simulink model "SST_MMC"  (R2014a)
settings: Solver=ode45  StartTime=0.0  StopTime=0.2  RelTol=1e-3
libraries: powerlib x328, simulink x1
(part 1 of 3)
settings Model: Creator=Shohag  LastModifiedBy=Shohag

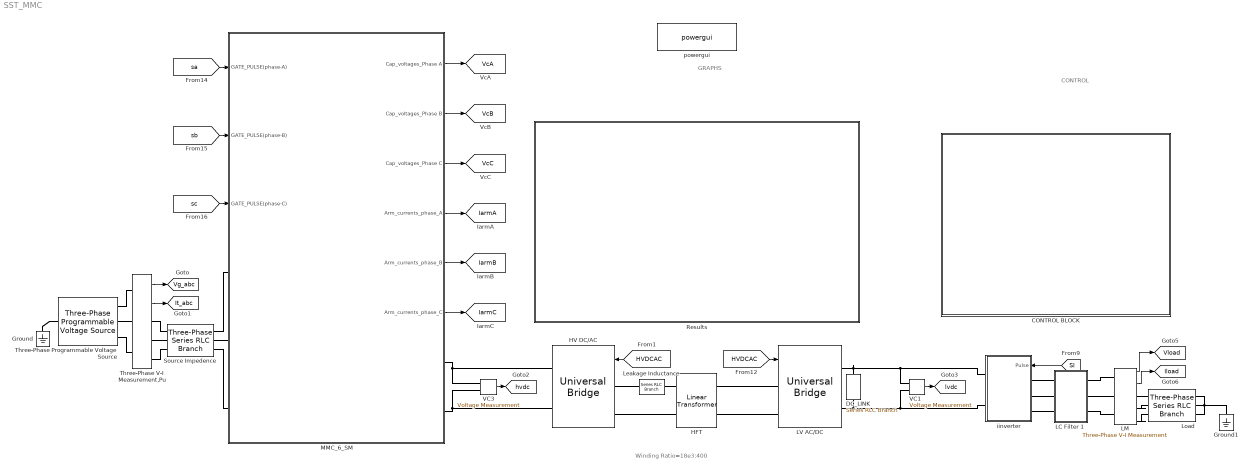
== system SST_MMC ==
  note: Winding Ratio=18e3:400
  note: GRAPHS
  note: CONTROL
  CONTROL BLOCK : Subsystem
  DC_LINK : powerlib/Elements/Series RLC Branch  LConnTagsString=__new0  RConnTagsString=__new0  BranchType=C  Resistance=1e3  Inductance=100e-6  SetiL0=off  InitialCurrent=0  Capacitance=1e-3  Setx0=off  InitialVoltage=415  Measurements=None
  Ground : powerlib/Elements/Ground  LConnTagsString=a
  Ground1 : powerlib/Elements/Ground  LConnTagsString=a
  HFT : powerlib/Elements/Linear Transformer  UNITS=pu  NominalPower=[ 10e3 10e3 ]  winding1="[ 18e3  0 0]"  winding2="[ 400  0 0]"  ThreeWindings=off  winding3=[ 315e3 0.002 0.08 ]  RmLm=[ 500e6 500e6 ]  Measurements=None  DataType=off
  HV DC/AC : powerlib/Power Electronics/Universal Bridge  Arms=2  SnubberResistance=1e5  SnubberCapacitance=inf  Device=IGBT / Diodes  Ron=1e-3  Lon=0  ForwardVoltages="[  0  0  ]"  ForwardVoltage=0  GTOparameters=[ 10e-6 , 20e-6 ]  IGBTparameters=[ 1e-6 , 2e-6 ]  Measurements=None  Measurements_2=None  converterType=Rectifier
  LC Filter 1 : Subsystem  mask{L=50e-3, C=100e-6}
      mask prompts: L "Inductance"; C "Capacitance"
  LM : powerlib/Measurements/Three-Phase V-I Measurement  VoltageMeasurement=phase-to-ground  SetLabelV=off  LabelV=Vabc  Vpu=off  VpuLL=off  CurrentMeasurement=yes  SetLabelI=off  LabelI=Iabc  Ipu=off  Pbase=20e6  Vbase=11e3  OutputType=Complex  PhasorSimulation=off  PSBequivalent=0
  LV AC/DC : powerlib/Power Electronics/Universal Bridge  Arms=2  SnubberResistance=1e5  SnubberCapacitance=inf  Device=IGBT / Diodes  Ron=1e-3  Lon=0  ForwardVoltages="[  0  0  ]"  ForwardVoltage=0  GTOparameters=[ 10e-6 , 20e-6 ]  IGBTparameters=[ 1e-6 , 2e-6 ]  Measurements=None  Measurements_2=None  converterType=Rectifier
  Leakage Inductance : powerlib/Elements/Series RLC Branch  LConnTagsString=__new0  RConnTagsString=__new0  BranchType=L  Resistance=1e3  Inductance=200e-6  SetiL0=off  InitialCurrent=0  Capacitance=0.001  Setx0=on  InitialVoltage=9e3  Measurements=None
  Load : powerlib/Elements/Three-Phase Series RLC Branch  LConnTagsString=A|B|C  RConnTagsString=A|B|C  BranchType=RL  Resistance=22  Inductance=10e-3  Capacitance=1e-6  Measurements=None
  MMC_6_SM : Subsystem  mask{C_SM=10e-3, VC_SM=3000, L_ARM=3e-3, Ron=1e-4}
      mask prompts: C_SM "Sub-module Capasitor Capasitance"; VC_SM "Sub-modue Capasitor Voltage"; L_ARM "Arm Inductance"
  Results : Subsystem
  Source Impedence : powerlib/Elements/Three-Phase Series RLC Branch  LConnTagsString=A|B|C  RConnTagsString=A|B|C  BranchType=RL  Resistance=0.5  Inductance=3e-3  Capacitance=1e-6  Measurements=None
  Three-Phase Programmable Voltage Source : powerlib/Electrical Sources/Three-Phase Programmable Voltage Source  PositiveSequence="[11e3  0 60]"  VariationEntity=Amplitude  VariationType=Table of time-amplitude pairs  VariationTypeAlt=Modulation  VariationStep=2  VariationRate=10  VariationMagnitude=0.3  VariationFrequency=5  VariationTiming=[0.1 0.2]  VariationPhaseA=on  Amplitudes=[1 0.8 1.2 0 0 1.2 1.0]  TimeValues=[0 0.03 0.05 0.07 0.08 0.09 0.1]  HarmonicGeneration=off  HarmonicA=[3 0.2 -25 0]  HarmonicB=[2 0.15 35 2]  Timing=[0.02 0.08]  BusType=PQ  Pref=10e3  Qref=0  Qmin=-inf  Qmax=inf
  Three-Phase V-I Measurement,Pu : powerlib/Measurements/Three-Phase V-I Measurement  VoltageMeasurement=phase-to-ground  SetLabelV=off  LabelV=Vabc  Vpu=off  VpuLL=off  CurrentMeasurement=yes  SetLabelI=off  LabelI=Iabc  Ipu=off  Pbase=20e6  Vbase=11e3  OutputType=Complex  PhasorSimulation=off  PSBequivalent=0
  VC1 : powerlib/Measurements/Voltage Measurement  PhasorSimulation=off  OutputType=Complex  PSBequivalent=0
  VC3 : powerlib/Measurements/Voltage Measurement  PhasorSimulation=off  OutputType=Complex  PSBequivalent=0
  iinverter : Subsystem
  powergui : powerlib/powergui  Priority=1  SimulationMode=Discrete  SolverType=Tustin  SampleTime=50e-6  frequency=60  SPID=on  DisableSnubberDevices=off  DisableRonSwitches=off  DisableVfSwitches=off  SwTol=0  Interpol=off  DisplayEquations=off  Ts=0  methode=off  frequencyindice=0  Pbase=100e6  ErrMax=1e-4  Iterations=50  UnitsV=kV  UnitsW=MW  FunctionMessages=off  echomessages=off  HookPort=off  EnableUseOfTLC=off  x0status=blocks  RestoreLinks=warning  ResistiveCurrentMeasurement=off  Frange=[0:2:500]  Ylog=off  Xlog=on  ShowGrid=off  save=off  variable=ZData  structure=0  ZoomFFT=off  StartTime=0.0  cycles=1  DisplayStyle=1  fundamental=60  FreqAxis=off  MaxFrequency=1000  frequencyindicesteady=1  RmsSteady=2  display=off
  tag scope: IarmA=global, IarmB=global, IarmC=global, Iload=global, It_abc=global, VcA=global, VcB=global, VcC=global, Vg_abc=global, Vload=global, hvdc=global, lvdc=global
  wires:
  MMC_6_SM/1(Cap_voltages_Phase A) -> [VcA]
  MMC_6_SM/2(Cap_voltages_Phase B) -> [VcB]
  MMC_6_SM/3(Cap_voltages_Phase C) -> [VcC]
  MMC_6_SM/4(Arm_currents_phase_A) -> [IarmA]
  MMC_6_SM/5(Arm_currents_phase_B) -> [IarmB]
  MMC_6_SM/6(Arm_currents_phase_C) -> [IarmC]
  Three-Phase V-I Measurement,Pu/1 -> [Vg_abc]
  Three-Phase V-I Measurement,Pu/2 -> [It_abc]
  VC3/1 -> [hvdc]
  [sa] -> MMC_6_SM/1(" GATE_PULSE(phase-A) ")
  [sb] -> MMC_6_SM/2(" GATE_PULSE(phase-B) ")
  [sc] -> MMC_6_SM/3(" GATE_PULSE(phase-C) ")
  VC1/1 -> [lvdc]
  [HVDCAC] -> HV DC/AC/1
  [HVDCAC] -> LV AC/DC/1
  [SI] -> iinverter/1(Pulse)
  LM/1 -> [Vload]
  LM/2 -> [Iload]
  connections:
  Source Impedence/RConn1 -- MMC_6_SM/LConn1
  Source Impedence/RConn2 -- MMC_6_SM/LConn2
  Three-Phase Programmable Voltage Source/RConn3 -- Three-Phase V-I Measurement,Pu/LConn3
  Three-Phase Programmable Voltage Source/RConn1 -- Three-Phase V-I Measurement,Pu/LConn1
  Three-Phase Programmable Voltage Source/RConn2 -- Three-Phase V-I Measurement,Pu/LConn2
  Three-Phase V-I Measurement,Pu/RConn3 -- Source Impedence/LConn3
  Three-Phase Programmable Voltage Source/LConn1 -- Ground/LConn1
  Three-Phase V-I Measurement,Pu/RConn1 -- Source Impedence/LConn1
  Source Impedence/RConn3 -- MMC_6_SM/LConn3
  Three-Phase V-I Measurement,Pu/RConn2 -- Source Impedence/LConn2
  HV DC/AC/LConn2 -- HFT/LConn2
  LV AC/DC/LConn1 -- HFT/RConn1
  LV AC/DC/LConn2 -- HFT/RConn2
  VC3/LConn2 -- HV DC/AC/RConn2 -- MMC_6_SM/RConn2
  HV DC/AC/LConn1 -- Leakage Inductance/RConn1
  VC1/LConn2 -- iinverter/RConn2 -- DC_LINK/RConn1 -- LV AC/DC/RConn2
  Leakage Inductance/LConn1 -- HFT/LConn1
  VC3/LConn1 -- HV DC/AC/RConn1 -- MMC_6_SM/RConn1
  VC1/LConn1 -- DC_LINK/LConn1 -- LV AC/DC/RConn1 -- iinverter/RConn1
  Load/RConn1 -- Ground1/LConn1 -- Load/RConn3 -- Load/RConn2
  LM/RConn1 -- Load/LConn1
  LM/RConn2 -- Load/LConn2
  LM/RConn3 -- Load/LConn3
  iinverter/LConn3 -- LC Filter 1/LConn3
  iinverter/LConn2 -- LC Filter 1/LConn2
  iinverter/LConn1 -- LC Filter 1/LConn1
  LC Filter 1/RConn1 -- LM/LConn1
  LC Filter 1/RConn2 -- LM/LConn2
  LC Filter 1/RConn3 -- LM/LConn3

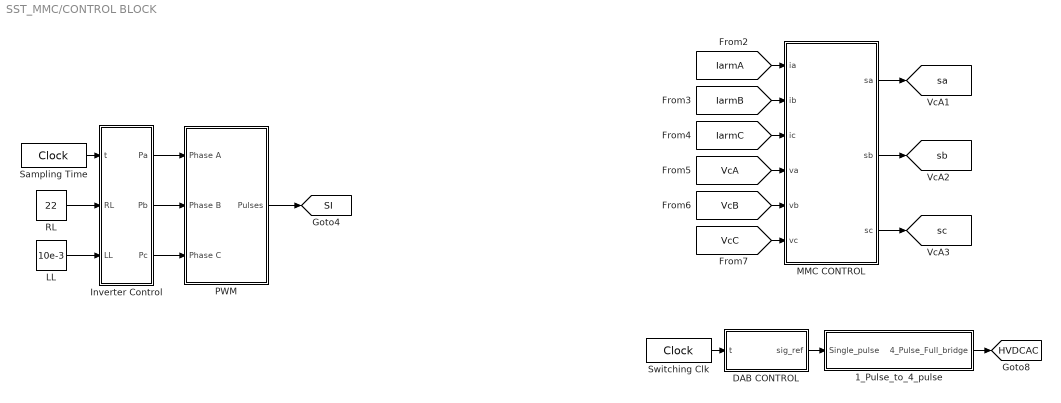
== system SST_MMC/CONTROL BLOCK ==
  1_Pulse_to_4_pulse : Subsystem
  DAB CONTROL : MATLAB Function  TreatAsAtomicUnit=on
  Inverter Control : MATLAB Function  TreatAsAtomicUnit=on
  LL : Constant  Value=10e-3
  MMC CONTROL : MATLAB Function  TreatAsAtomicUnit=on
  PWM : Subsystem  mask{Fs=10e3}
      mask prompts: Fs "Frequency"
  RL : Constant  Value=22
  Sampling Time : DigitalClock  SampleTime=100e-6
  Switching Clk : DigitalClock  SampleTime=5e-5
  tag scope: HVDCAC=global, SI=global, sa=global, sb=global, sc=global
  wires:
  LL/1 -> Inverter Control/3(LL)
  RL/1 -> Inverter Control/2(RL)
  Inverter Control/1(Pa) -> PWM/1(Phase A)
  Inverter Control/2(Pb) -> PWM/2(Phase B)
  Inverter Control/3(Pc) -> PWM/3(Phase C)
  PWM/1(Pulses) -> [SI]
  Switching Clk/1 -> DAB CONTROL/1(t)
  MMC CONTROL/3(sc) -> [sc]
  MMC CONTROL/2(sb) -> [sb]
  MMC CONTROL/1(sa) -> [sa]
  1_Pulse_to_4_pulse/1(4_Pulse_Full_bridge) -> [HVDCAC]
  DAB CONTROL/1(sig_ref) -> 1_Pulse_to_4_pulse/1(Single_pulse)
  Sampling Time/1 -> Inverter Control/1(t)
  [VcA] -> MMC CONTROL/4(va)
  [IarmC] -> MMC CONTROL/3(ic)
  [IarmB] -> MMC CONTROL/2(ib)
  [VcC] -> MMC CONTROL/6(vc)
  [IarmA] -> MMC CONTROL/1(ia)
  [VcB] -> MMC CONTROL/5(vb)

== system SST_MMC/LC Filter 1 ==
  C5 : powerlib/Elements/Parallel RLC Branch  LConnTagsString=a  RConnTagsString=__new0  BranchType=C  Resistance=inf  Inductance=inf  SetiL0=off  InitialCurrent=0  Capacitance=C  Setx0=off  InitialVoltage=0  Measurements=None
  C6 : powerlib/Elements/Parallel RLC Branch  LConnTagsString=a  RConnTagsString=__new0  BranchType=C  Resistance=inf  Inductance=inf  SetiL0=off  InitialCurrent=0  Capacitance=C  Setx0=off  InitialVoltage=0  Measurements=None
  C7 : powerlib/Elements/Parallel RLC Branch  LConnTagsString=a  RConnTagsString=__new0  BranchType=C  Resistance=inf  Inductance=inf  SetiL0=off  InitialCurrent=0  Capacitance=C  Setx0=off  InitialVoltage=0  Measurements=None
  Ground2 : powerlib/Elements/Ground  LConnTagsString=a
  L4 : powerlib/Elements/Parallel RLC Branch  LConnTagsString=a  RConnTagsString=__new0  BranchType=L  Resistance=inf  Inductance=L  SetiL0=off  InitialCurrent=0  Capacitance=1.3e-3  Setx0=off  InitialVoltage=0  Measurements=None
  L5 : powerlib/Elements/Parallel RLC Branch  LConnTagsString=a  RConnTagsString=__new0  BranchType=L  Resistance=inf  Inductance=L  SetiL0=off  InitialCurrent=0  Capacitance=1.3e-3  Setx0=off  InitialVoltage=0  Measurements=None
  L6 : powerlib/Elements/Parallel RLC Branch  LConnTagsString=a  RConnTagsString=__new0  BranchType=L  Resistance=inf  Inductance=L  SetiL0=off  InitialCurrent=0  Capacitance=1.3e-3  Setx0=off  InitialVoltage=0  Measurements=None
  A : PMIOPort  Port=1  Side=Left
  A1 : PMIOPort  Port=2  Side=Right
  B : PMIOPort  Port=3  Side=Left
  B1 : PMIOPort  Port=4  Side=Right
  C1 : PMIOPort  Port=5  Side=Right
  C : PMIOPort  Port=6  Side=Left
  connections:
  L4/LConn1 -- A/RConn1
  L6/LConn1 -- C/RConn1
  C5/RConn1 -- C7/RConn1 -- Ground2/LConn1 -- C6/RConn1
  L5/LConn1 -- B/RConn1
  C6/LConn1 -- B1/RConn1 -- L5/RConn1
  L4/RConn1 -- A1/RConn1 -- C5/LConn1
  C7/LConn1 -- C1/RConn1 -- L6/RConn1

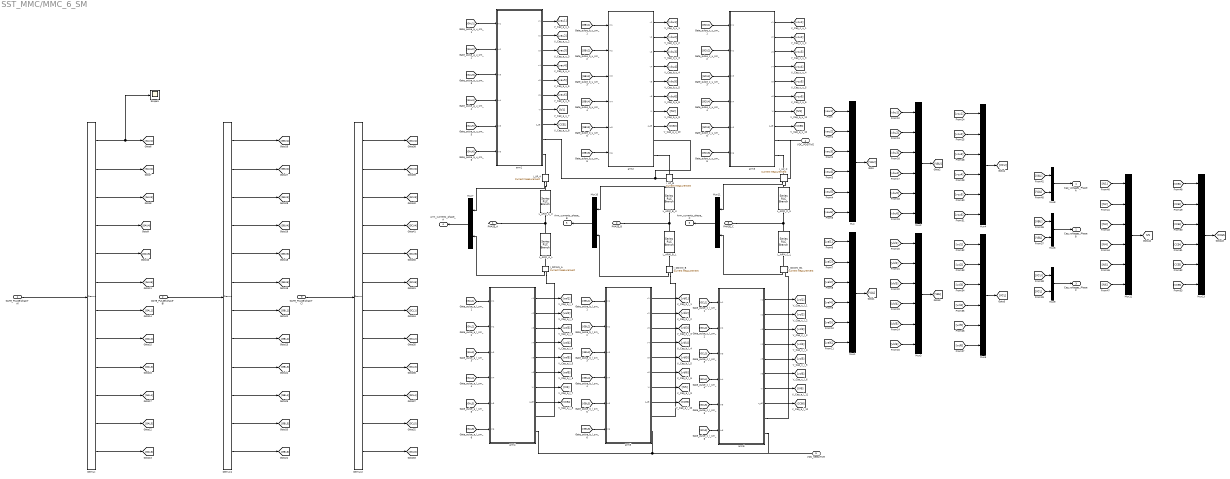
== system SST_MMC/MMC_6_SM ==
  " GATE_PULSE(phase-A) " : Inport
  " GATE_PULSE(phase-B) " : Inport  Port=2
  " GATE_PULSE(phase-C) " : Inport  Port=3
  Demux : Demux  Outputs=12
  Demux1 : Demux  Outputs=12
  Demux2 : Demux  Outputs=12
  I_DOWN_A : powerlib/Measurements/Current Measurement  PhasorSimulation=off  OutputType=Complex  PSBequivalent=0
  I_DOWN_B : powerlib/Measurements/Current Measurement  PhasorSimulation=off  OutputType=Complex  PSBequivalent=0
  I_DOWN_B1 : powerlib/Measurements/Current Measurement  PhasorSimulation=off  OutputType=Complex  PSBequivalent=0
  I_UP_A : powerlib/Measurements/Current Measurement  PhasorSimulation=off  OutputType=Complex  PSBequivalent=0
  I_UP_B : powerlib/Measurements/Current Measurement  PhasorSimulation=off  OutputType=Complex  PSBequivalent=0
  I_UP_C : powerlib/Measurements/Current Measurement  PhasorSimulation=off  OutputType=Complex  PSBequivalent=0
  L_ARM_A_L : powerlib/Elements/Series RLC Branch  LConnTagsString=__new0  RConnTagsString=__new0  BranchType=L  Resistance=1  Inductance=L_ARM  SetiL0=off  InitialCurrent=0  Capacitance=1e-6  Setx0=off  InitialVoltage=0  Measurements=None
  L_ARM_A_U : powerlib/Elements/Series RLC Branch  LConnTagsString=__new0  RConnTagsString=__new0  BranchType=L  Resistance=1  Inductance=L_ARM  SetiL0=off  InitialCurrent=0  Capacitance=1e-6  Setx0=off  InitialVoltage=0  Measurements=None
  L_ARM_B_L : powerlib/Elements/Series RLC Branch  LConnTagsString=__new0  RConnTagsString=__new0  BranchType=L  Resistance=1  Inductance=L_ARM  SetiL0=off  InitialCurrent=0  Capacitance=1e-6  Setx0=off  InitialVoltage=0  Measurements=None
  L_ARM_B_U : powerlib/Elements/Series RLC Branch  LConnTagsString=__new0  RConnTagsString=__new0  BranchType=L  Resistance=1  Inductance=L_ARM  SetiL0=off  InitialCurrent=0  Capacitance=1e-6  Setx0=off  InitialVoltage=0  Measurements=None
  L_ARM_C_L : powerlib/Elements/Series RLC Branch  LConnTagsString=__new0  RConnTagsString=__new0  BranchType=L  Resistance=1  Inductance=L_ARM  SetiL0=off  InitialCurrent=0  Capacitance=1e-6  Setx0=off  InitialVoltage=0  Measurements=None
  L_ARM_C_U : powerlib/Elements/Series RLC Branch  LConnTagsString=__new0  RConnTagsString=__new0  BranchType=L  Resistance=1  Inductance=L_ARM  SetiL0=off  InitialCurrent=0  Capacitance=1e-6  Setx0=off  InitialVoltage=0  Measurements=None
  Mux{,1..5,12..13} (8 alike) : Mux  Inputs=6
  Mux{6..11} (6 alike) : Mux  Inputs=2
  Scope1 : Scope
      settings: YMin=0.95  YMax=1.05  SaveName=ScopeData3
  arm1 : Subsystem
  arm2 : Subsystem
  arm3 : Subsystem
  arm4 : Subsystem
  arm5 : Subsystem
  arm6 : Subsystem
  PHASE_A : PMIOPort  Port=1  Side=Left
  PHASE_B : PMIOPort  Port=2  Side=Left
  PHASE_C : PMIOPort  Port=3  Side=Left
  VDC_POSITIVE : PMIOPort  Port=4  Side=Right
  VDC_NEGATIVE : PMIOPort  Port=5  Side=Right
  Cap_voltages_Phase A : Outport
  Cap_voltages_Phase B : Outport  Port=2
  Cap_voltages_Phase C : Outport  Port=3
  Arm_currents_phase_A : Outport  Port=4
  Arm_currents_phase_B : Outport  Port=5
  Arm_currents_phase_C : Outport  Port=6
  tag scope: CCES=global, IVS=global
  wires:
  Demux/4 -> [GAU4]
  Demux/2 -> [GAU2]
  [vau2] -> Mux/2
  [vau1] -> Mux/1
  Mux/1 -> [VAU]
  Demux/1 -> Scope1/1, [GAU1]
  [vbl6] -> Mux3/6
  [vbl4] -> Mux3/4
  [vbu6] -> Mux2/6
  [vbu1] -> Mux2/1
  [vbu4] -> Mux2/4
  [vbl3] -> Mux3/3
  Mux2/1 -> [VBU]
  [vbu3] -> Mux2/3
  [vbl1] -> Mux3/1
  Mux3/1 -> [VBL]
  [vbu5] -> Mux2/5
  [vbu2] -> Mux2/2
  [vbl2] -> Mux3/2
  [vbl5] -> Mux3/5
  Demux1/1 -> [GBU1]
  Demux1/3 -> [GBU3]
  [vcl6] -> Mux5/6
  [vcl5] -> Mux5/5
  [vcu3] -> Mux4/3
  [vcl1] -> Mux5/1
  [vcl4] -> Mux5/4
  [vcu5] -> Mux4/5
  [vcu2] -> Mux4/2
  [vcl3] -> Mux5/3
  Mux4/1 -> [VCU]
  [vcu6] -> Mux4/6
  Mux5/1 -> [VCL]
  [vcl2] -> Mux5/2
  [vcu1] -> Mux4/1
  [vcu4] -> Mux4/4
  [vau3] -> Mux/3
  [val5] -> Mux1/5
  Demux/3 -> [GAU3]
  Demux/5 -> [GAU5]
  [vau6] -> Mux/6
  [val4] -> Mux1/4
  Mux1/1 -> [VAL]
  [vau4] -> Mux/4
  [val3] -> Mux1/3
  [val6] -> Mux1/6
  [val2] -> Mux1/2
  Demux/6 -> [GAU6]
  [vau5] -> Mux/5
  [val1] -> Mux1/1
  Mux7/1 -> Arm_currents_phase_A/1
  [VAL] -> Mux8/2
  [VAU] -> Mux8/1
  Mux8/1 -> Cap_voltages_Phase A/1
  Demux/7 -> [GAL1]
  Demux/8 -> [GAL2]
  Demux/9 -> [GAL3]
  Demux/10 -> [GAL4]
  Demux/11 -> [GAL5]
  Demux/12 -> [GAL6]
  Demux1/2 -> [GBU2]
  Demux1/4 -> [GBU4]
  Demux1/5 -> [GBU5]
  Demux1/6 -> [GBU6]
  Demux1/7 -> [GBL1]
  Demux1/8 -> [GBL2]
  Demux1/9 -> [GBL3]
  Demux1/10 -> [GBL4]
  Demux1/11 -> [GBL5]
  Demux1/12 -> [GBL6]
  Demux2/1 -> [GCU1]
  Demux2/2 -> [GCU2]
  Demux2/3 -> [GCU3]
  Demux2/4 -> [GCU4]
  Demux2/5 -> [GCU5]
  Demux2/6 -> [GCU6]
  Demux2/7 -> [GCL1]
  Demux2/8 -> [GCL2]
  Demux2/9 -> [GCL3]
  Demux2/10 -> [GCL4]
  Demux2/11 -> [GCL5]
  Demux2/12 -> [GCL6]
  [VBL] -> Mux6/2
  [VBU] -> Mux6/1
  Mux6/1 -> Cap_voltages_Phase B/1
  [VCL] -> Mux9/2
  [VCU] -> Mux9/1
  Mux9/1 -> Cap_voltages_Phase C/1
  Mux10/1 -> Arm_currents_phase_B/1
  I_DOWN_B/1 -> Mux10/2
  Mux11/1 -> Arm_currents_phase_C/1
  I_DOWN_B1/1 -> Mux11/2
  I_UP_A/1 -> Mux7/1
  I_DOWN_A/1 -> Mux7/2
  I_UP_B/1 -> Mux10/1
  I_UP_C/1 -> Mux11/1
  " GATE_PULSE(phase-A) "/1 -> Demux/1
  " GATE_PULSE(phase-B) "/1 -> Demux1/1
  " GATE_PULSE(phase-C) "/1 -> Demux2/1
  [GAU6] -> arm1/6(In6)
  [GAU5] -> arm1/5(In5)
  [GAU4] -> arm1/4(In4)
  [GAU3] -> arm1/3(In3)
  [GAU2] -> arm1/2(In2)
  [GAU1] -> arm1/1(In1)
  arm1/1(v1) -> [vau1]
  arm1/2(v2) -> [vau2]
  arm1/3(v3) -> [vau3]
  arm1/4(v4) -> [vau4]
  arm1/5(v5) -> [vau5]
  arm1/6(v6) -> [vau6]
  [GBU6] -> arm2/6(In6)
  [GBU5] -> arm2/5(In5)
  [GBU4] -> arm2/4(In4)
  [GBU3] -> arm2/3(In3)
  [GBU2] -> arm2/2(In2)
  [GBU1] -> arm2/1(In1)
  arm2/1(v1) -> [vbu1]
  arm2/2(v2) -> [vbu2]
  arm2/3(v3) -> [vbu3]
  arm2/4(v4) -> [vbu4]
  arm2/5(v5) -> [vbu5]
  arm2/6(v6) -> [vbu6]
  arm1/7(VI) -> [IV1]
  arm1/8(c_cE) -> [CCE1]
  arm2/7(VI) -> [IV2]
  arm2/8(c_cE) -> [CCE2]
  [GCU6] -> arm3/6(In6)
  [GCU5] -> arm3/5(In5)
  [GCU4] -> arm3/4(In4)
  [GCU3] -> arm3/3(In3)
  [GCU2] -> arm3/2(In2)
  [GCU1] -> arm3/1(In1)
  arm3/1(v1) -> [vcu1]
  arm3/2(v2) -> [vcu2]
  arm3/3(v3) -> [vcu3]
  arm3/4(v4) -> [vcu4]
  arm3/5(v5) -> [vcu5]
  arm3/6(v6) -> [vcu6]
  arm3/7(VI) -> [IV3]
  arm3/8(c_cE) -> [CCE3]
  [GAL1] -> arm4/1(In1)
  [GAL2] -> arm4/2(In2)
  [GAL3] -> arm4/3(In3)
  [GAL4] -> arm4/4(In4)
  [GAL5] -> arm4/5(In5)
  [GAL6] -> arm4/6(In6)
  arm4/1(v1) -> [val1]
  arm4/2(v2) -> [val2]
  arm4/3(v3) -> [val3]
  arm4/4(v4) -> [val4]
  arm4/5(v5) -> [val5]
  arm4/6(v6) -> [val6]
  arm4/7(VI) -> [IV4]
  arm4/8(c_cE) -> [CCE4]
  [GBL1] -> arm5/1(In1)
  [GBL2] -> arm5/2(In2)
  [GBL3] -> arm5/3(In3)
  [GBL4] -> arm5/4(In4)
  [GBL5] -> arm5/5(In5)
  [GBL6] -> arm5/6(In6)
  arm5/1(v1) -> [vbl1]
  arm5/2(v2) -> [vbl2]
  arm5/3(v3) -> [vbl3]
  arm5/4(v4) -> [vbl4]
  arm5/5(v5) -> [vbl5]
  arm5/6(v6) -> [vbl6]
  arm5/7(VI) -> [IV5]
  arm5/8(c_cE) -> [CCE5]
  [GCL1] -> arm6/1(In1)
  [GCL2] -> arm6/2(In2)
  [GCL3] -> arm6/3(In3)
  [GCL4] -> arm6/4(In4)
  [GCL5] -> arm6/5(In5)
  [GCL6] -> arm6/6(In6)
  arm6/1(v1) -> [vcl1]
  arm6/2(v2) -> [vcl2]
  arm6/3(v3) -> [vcl3]
  arm6/4(v4) -> [vcl4]
  arm6/5(v5) -> [vcl5]
  arm6/6(v6) -> [vcl6]
  arm6/7(VI) -> [IV6]
  arm6/8(c_cE) -> [CCE6]
  [IV5] -> Mux12/5
  [IV2] -> Mux12/2
  Mux12/1 -> [IVS]
  [IV6] -> Mux12/6
  [IV1] -> Mux12/1
  [IV4] -> Mux12/4
  [CCE3] -> Mux13/3
  [CCE5] -> Mux13/5
  [CCE2] -> Mux13/2
  Mux13/1 -> [CCES]
  [CCE6] -> Mux13/6
  [CCE1] -> Mux13/1
  [CCE4] -> Mux13/4
  [IV3] -> Mux12/3
  connections:
  L_ARM_A_U/RConn1 -- PHASE_A/RConn1 -- L_ARM_A_L/LConn1
  L_ARM_B_U/RConn1 -- PHASE_B/RConn1 -- L_ARM_B_L/LConn1
  L_ARM_C_U/RConn1 -- PHASE_C/RConn1 -- L_ARM_C_L/LConn1
  L_ARM_B_L/RConn1 -- I_DOWN_B/LConn1
  L_ARM_C_L/RConn1 -- I_DOWN_B1/LConn1
  I_UP_A/RConn1 -- L_ARM_A_U/LConn1
  I_DOWN_A/LConn1 -- L_ARM_A_L/RConn1
  I_UP_B/RConn1 -- L_ARM_B_U/LConn1
  I_UP_C/RConn1 -- L_ARM_C_U/LConn1
  arm1/RConn1 -- arm2/RConn1 -- VDC_POSITIVE/RConn1 -- arm3/RConn1
  I_DOWN_A/RConn1 -- arm4/RConn1
  I_DOWN_B/RConn1 -- arm5/RConn1
  arm4/RConn2 -- arm6/RConn2 -- VDC_NEGATIVE/RConn1 -- arm5/RConn2
  arm6/RConn1 -- I_DOWN_B1/RConn1
  arm1/RConn2 -- I_UP_A/LConn1
  arm2/RConn2 -- I_UP_B/LConn1
  arm3/RConn2 -- I_UP_C/LConn1

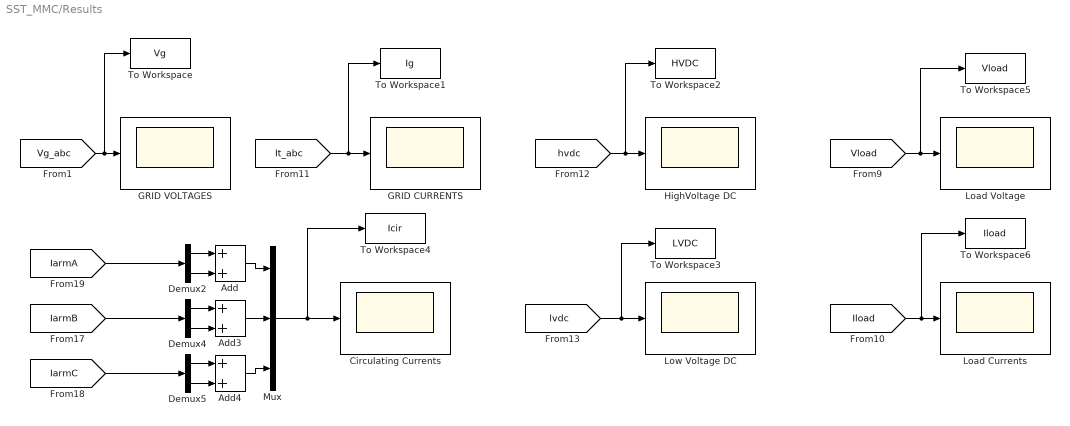
== system SST_MMC/Results ==
  Add : Sum
  Add3 : Sum
  Add4 : Sum
  Circulating Currents : Scope
      settings: YMin=-30  YMax=40  SaveName=ScopeData5
  Demux2 : Demux  Outputs=2
  Demux4 : Demux  Outputs=2
  Demux5 : Demux  Outputs=2
  GRID CURRENTS : Scope
      settings: YMin=-20000  YMax=20000  SaveName=ScopeData4
  GRID VOLTAGES : Scope
      settings: YMin=-17500  YMax=17500
  HighVoltage DC : Scope
      settings: YMin=15500  YMax=20500  SaveName=ScopeData6
  Load Currents : Scope
      settings: YMin=-25  YMax=35  SaveName=ScopeData10
  Load Voltage : Scope
      settings: YMin=-300  YMax=300  SaveName=ScopeData9
  Low Voltage DC : Scope
      settings: YMin=427.75  YMax=432.25  SaveName=ScopeData8
  Mux : Mux  Inputs=3
  To Workspace : ToWorkspace  VariableName=Vg  SaveFormat=Timeseries  SampleTime=-1
  To Workspace1 : ToWorkspace  VariableName=Ig  SaveFormat=Timeseries  SampleTime=-1
  To Workspace2 : ToWorkspace  VariableName=HVDC  SaveFormat=Timeseries  SampleTime=-1
  To Workspace3 : ToWorkspace  VariableName=LVDC  SaveFormat=Timeseries  SampleTime=-1
  To Workspace4 : ToWorkspace  VariableName=Icir  SaveFormat=Timeseries  SampleTime=-1
  To Workspace5 : ToWorkspace  VariableName=Vload  SaveFormat=Timeseries  SampleTime=-1
  To Workspace6 : ToWorkspace  VariableName=Iload  SaveFormat=Timeseries  SampleTime=-1
  wires:
  [hvdc] -> To Workspace2/1, HighVoltage DC/1
  Add4/1 -> Mux/3
  [IarmA] -> Demux2/1
  Demux2/1 -> Add/1
  Demux2/2 -> Add/2
  [Vg_abc] -> To Workspace/1, GRID VOLTAGES/1
  Demux4/2 -> Add3/2
  [IarmB] -> Demux4/1
  Demux5/1 -> Add4/1
  Mux/1 -> To Workspace4/1, Circulating Currents/1
  Add3/1 -> Mux/2
  Demux5/2 -> Add4/2
  Add/1 -> Mux/1
  [lvdc] -> To Workspace3/1, Low Voltage DC/1
  Demux4/1 -> Add3/1
  [IarmC] -> Demux5/1
  [It_abc] -> To Workspace1/1, GRID CURRENTS/1
  [Vload] -> To Workspace5/1, Load Voltage/1
  [Iload] -> To Workspace6/1, Load Currents/1

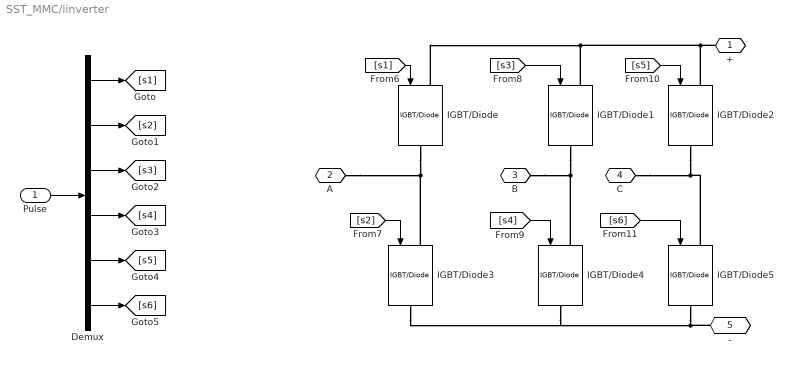
== system SST_MMC/iinverter ==
  Pulse : Inport
  Demux : Demux  Outputs=6
  IGBT/Diode{,1..5} (6 alike) : powerlib/Power Electronics/IGBT//Diode  Ron=1e-3  Rs=1e5  Cs=inf  Measurements=off
  + : PMIOPort  Port=1  Side=Right
  A : PMIOPort  Port=2  Side=Left
  B : PMIOPort  Port=3  Side=Left
  C : PMIOPort  Port=4  Side=Left
  - : PMIOPort  Port=5  Side=Right
  wires:
  [s1] -> IGBT/Diode/1
  [s2] -> IGBT/Diode3/1
  [s3] -> IGBT/Diode1/1
  [s4] -> IGBT/Diode4/1
  [s5] -> IGBT/Diode2/1
  [s6] -> IGBT/Diode5/1
  Demux/1 -> [s1]
  Demux/2 -> [s2]
  Demux/3 -> [s3]
  Demux/4 -> [s4]
  Demux/5 -> [s5]
  Demux/6 -> [s6]
  Pulse/1 -> Demux/1
  connections:
  +/RConn1 -- IGBT/Diode/LConn1 -- IGBT/Diode1/LConn1 -- IGBT/Diode2/LConn1
  IGBT/Diode4/RConn1 -- IGBT/Diode3/RConn1 -- IGBT/Diode5/RConn1 -- -/RConn1
  A/RConn1 -- IGBT/Diode3/LConn1 -- IGBT/Diode/RConn1
  B/RConn1 -- IGBT/Diode4/LConn1 -- IGBT/Diode1/RConn1
  C/RConn1 -- IGBT/Diode5/LConn1 -- IGBT/Diode2/RConn1

== system SST_MMC/CONTROL BLOCK/1_Pulse_to_4_pulse ==
  Single_pulse : Inport
  Mux1 : Mux
  Relay4 : Relay
  Relay5 : Relay  OnOutputValue=0  OffOutputValue=1
  Relay6 : Relay  OnOutputValue=0  OffOutputValue=1
  Relay7 : Relay
  4_Pulse_Full_bridge : Outport
  wires:
  Single_pulse/1 -> Relay5/1, Relay4/1, Relay7/1, Relay6/1
  Mux1/1 -> 4_Pulse_Full_bridge/1
  Relay6/1 -> Mux1/3
  Relay4/1 -> Mux1/1
  Relay7/1 -> Mux1/4
  Relay5/1 -> Mux1/2

== system SST_MMC/CONTROL BLOCK/PWM ==
  Phase A : Inport
  Phase B : Inport  Port=2
  Phase C : Inport  Port=3
  BL1 : Logic  Operator=NOT  Inputs=1
  BL2 : Logic  Operator=NOT  Inputs=1
  BL5 : Logic  Operator=NOT  Inputs=1
  Mux : Mux  Inputs=6
  Relational Operator1 : RelationalOperator  Operator=<=
  Relational Operator2 : RelationalOperator  Operator=<=
  Relational Operator3 : RelationalOperator  Operator=<=
  Triangle : simulink/Sources/Repeating Sequence  rep_seq_t=[0 1/Fs/4 3/Fs/4 1/Fs]  rep_seq_y=[0 -1 1 0]
  Pulses : Outport
  wires:
  Relational Operator3/1 -> Mux/5, BL2/1
  Triangle/1 -> Relational Operator3/1, Relational Operator1/1, Relational Operator2/1
  BL2/1 -> Mux/6
  BL5/1 -> Mux/2
  Mux/1 -> Pulses/1
  Relational Operator2/1 -> Mux/1, BL5/1
  Relational Operator1/1 -> Mux/3, BL1/1
  Phase C/1 -> Relational Operator3/2
  Phase A/1 -> Relational Operator2/2
  Phase B/1 -> Relational Operator1/2
  BL1/1 -> Mux/4

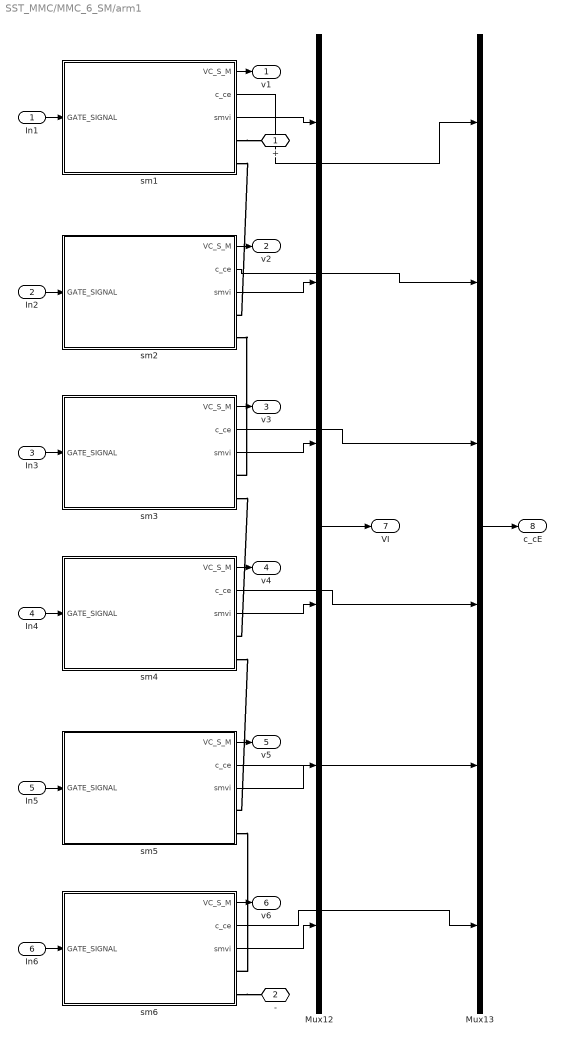
== system SST_MMC/MMC_6_SM/arm1 ==
  In1 : Inport
  In2 : Inport  Port=2
  In3 : Inport  Port=3
  In4 : Inport  Port=4
  In5 : Inport  Port=5
  In6 : Inport  Port=6
  Mux12 : Mux  Inputs=6
  Mux13 : Mux  Inputs=6
  sm1 : Subsystem
  sm2 : Subsystem
  sm3 : Subsystem
  sm4 : Subsystem
  sm5 : Subsystem
  sm6 : Subsystem
  + : PMIOPort  Port=1  Side=Right
  - : PMIOPort  Port=2  Side=Right
  v1 : Outport
  v2 : Outport  Port=2
  v3 : Outport  Port=3
  v4 : Outport  Port=4
  v5 : Outport  Port=5
  v6 : Outport  Port=6
  VI : Outport  Port=7
  c_cE : Outport  Port=8
  wires:
  sm4/2(" c_ce") -> Mux13/4
  sm5/3(" smvi") -> Mux12/5
  sm3/1(" VC_S_M") -> v3/1
  Mux13/1 -> c_cE/1
  In5/1 -> sm5/1(" GATE_SIGNAL ")
  In4/1 -> sm4/1(" GATE_SIGNAL ")
  sm5/1(" VC_S_M") -> v5/1
  In3/1 -> sm3/1(" GATE_SIGNAL ")
  sm6/1(" VC_S_M") -> v6/1
  In2/1 -> sm2/1(" GATE_SIGNAL ")
  sm2/3(" smvi") -> Mux12/2
  In1/1 -> sm1/1(" GATE_SIGNAL ")
  sm2/1(" VC_S_M") -> v2/1
  In6/1 -> sm6/1(" GATE_SIGNAL ")
  sm4/3(" smvi") -> Mux12/4
  sm1/1(" VC_S_M") -> v1/1
  sm4/1(" VC_S_M") -> v4/1
  Mux12/1 -> VI/1
  sm5/2(" c_ce") -> Mux13/5
  sm6/3(" smvi") -> Mux12/6
  sm3/2(" c_ce") -> Mux13/3
  sm1/2(" c_ce") -> Mux13/1
  sm2/2(" c_ce") -> Mux13/2
  sm3/3(" smvi") -> Mux12/3
  sm6/2(" c_ce") -> Mux13/6
  sm1/3(" smvi") -> Mux12/1
  connections:
  sm6/RConn2 -- -/RConn1
  sm1/RConn2 -- sm2/RConn1
  sm1/RConn1 -- +/RConn1
  sm2/RConn2 -- sm3/RConn1
  sm4/RConn2 -- sm5/RConn1
  sm5/RConn2 -- sm6/RConn1
  sm3/RConn2 -- sm4/RConn1

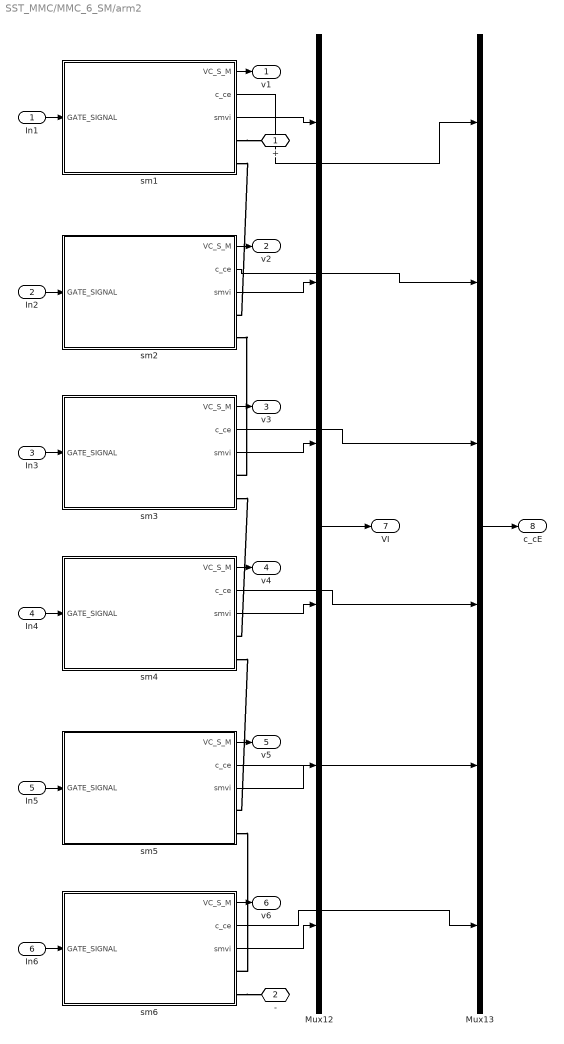
== system SST_MMC/MMC_6_SM/arm2 ==
  In1 : Inport
  In2 : Inport  Port=2
  In3 : Inport  Port=3
  In4 : Inport  Port=4
  In5 : Inport  Port=5
  In6 : Inport  Port=6
  Mux12 : Mux  Inputs=6
  Mux13 : Mux  Inputs=6
  sm1 : Subsystem
  sm2 : Subsystem
  sm3 : Subsystem
  sm4 : Subsystem
  sm5 : Subsystem
  sm6 : Subsystem
  + : PMIOPort  Port=1  Side=Right
  - : PMIOPort  Port=2  Side=Right
  v1 : Outport
  v2 : Outport  Port=2
  v3 : Outport  Port=3
  v4 : Outport  Port=4
  v5 : Outport  Port=5
  v6 : Outport  Port=6
  VI : Outport  Port=7
  c_cE : Outport  Port=8
  wires:
  sm1/3(" smvi") -> Mux12/1
  sm6/2(" c_ce") -> Mux13/6
  sm3/3(" smvi") -> Mux12/3
  sm2/2(" c_ce") -> Mux13/2
  sm1/2(" c_ce") -> Mux13/1
  sm3/2(" c_ce") -> Mux13/3
  sm6/3(" smvi") -> Mux12/6
  sm5/2(" c_ce") -> Mux13/5
  Mux12/1 -> VI/1
  sm4/1(" VC_S_M") -> v4/1
  sm1/1(" VC_S_M") -> v1/1
  sm4/3(" smvi") -> Mux12/4
  In6/1 -> sm6/1(" GATE_SIGNAL ")
  sm2/1(" VC_S_M") -> v2/1
  In1/1 -> sm1/1(" GATE_SIGNAL ")
  sm2/3(" smvi") -> Mux12/2
  In2/1 -> sm2/1(" GATE_SIGNAL ")
  sm6/1(" VC_S_M") -> v6/1
  In3/1 -> sm3/1(" GATE_SIGNAL ")
  sm5/1(" VC_S_M") -> v5/1
  In4/1 -> sm4/1(" GATE_SIGNAL ")
  In5/1 -> sm5/1(" GATE_SIGNAL ")
  Mux13/1 -> c_cE/1
  sm3/1(" VC_S_M") -> v3/1
  sm5/3(" smvi") -> Mux12/5
  sm4/2(" c_ce") -> Mux13/4
  connections:
  sm3/RConn2 -- sm4/RConn1
  sm5/RConn2 -- sm6/RConn1
  sm4/RConn2 -- sm5/RConn1
  sm2/RConn2 -- sm3/RConn1
  sm1/RConn1 -- +/RConn1
  sm1/RConn2 -- sm2/RConn1
  sm6/RConn2 -- -/RConn1

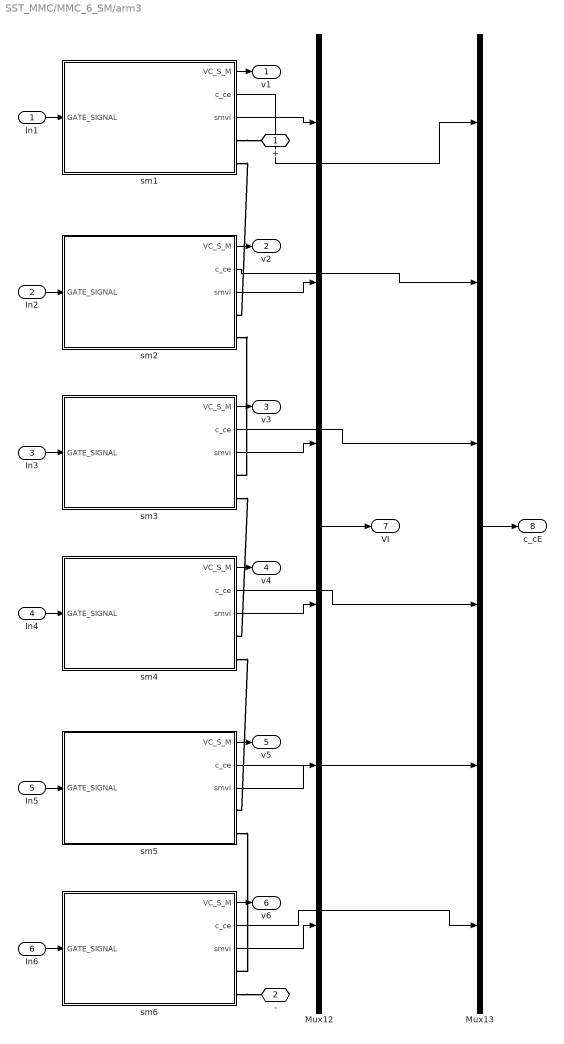
== system SST_MMC/MMC_6_SM/arm3 ==
  In1 : Inport
  In2 : Inport  Port=2
  In3 : Inport  Port=3
  In4 : Inport  Port=4
  In5 : Inport  Port=5
  In6 : Inport  Port=6
  Mux12 : Mux  Inputs=6
  Mux13 : Mux  Inputs=6
  sm1 : Subsystem
  sm2 : Subsystem
  sm3 : Subsystem
  sm4 : Subsystem
  sm5 : Subsystem
  sm6 : Subsystem
  + : PMIOPort  Port=1  Side=Right
  - : PMIOPort  Port=2  Side=Right
  v1 : Outport
  v2 : Outport  Port=2
  v3 : Outport  Port=3
  v4 : Outport  Port=4
  v5 : Outport  Port=5
  v6 : Outport  Port=6
  VI : Outport  Port=7
  c_cE : Outport  Port=8
  wires:
  sm4/2(" c_ce") -> Mux13/4
  sm5/3(" smvi") -> Mux12/5
  sm3/1(" VC_S_M") -> v3/1
  Mux13/1 -> c_cE/1
  In5/1 -> sm5/1(" GATE_SIGNAL ")
  In4/1 -> sm4/1(" GATE_SIGNAL ")
  sm5/1(" VC_S_M") -> v5/1
  In3/1 -> sm3/1(" GATE_SIGNAL ")
  sm6/1(" VC_S_M") -> v6/1
  In2/1 -> sm2/1(" GATE_SIGNAL ")
  sm2/3(" smvi") -> Mux12/2
  In1/1 -> sm1/1(" GATE_SIGNAL ")
  sm2/1(" VC_S_M") -> v2/1
  In6/1 -> sm6/1(" GATE_SIGNAL ")
  sm4/3(" smvi") -> Mux12/4
  sm1/1(" VC_S_M") -> v1/1
  sm4/1(" VC_S_M") -> v4/1
  Mux12/1 -> VI/1
  sm5/2(" c_ce") -> Mux13/5
  sm6/3(" smvi") -> Mux12/6
  sm3/2(" c_ce") -> Mux13/3
  sm1/2(" c_ce") -> Mux13/1
  sm2/2(" c_ce") -> Mux13/2
  sm3/3(" smvi") -> Mux12/3
  sm6/2(" c_ce") -> Mux13/6
  sm1/3(" smvi") -> Mux12/1
  connections:
  sm6/RConn2 -- -/RConn1
  sm1/RConn2 -- sm2/RConn1
  sm1/RConn1 -- +/RConn1
  sm2/RConn2 -- sm3/RConn1
  sm4/RConn2 -- sm5/RConn1
  sm5/RConn2 -- sm6/RConn1
  sm3/RConn2 -- sm4/RConn1

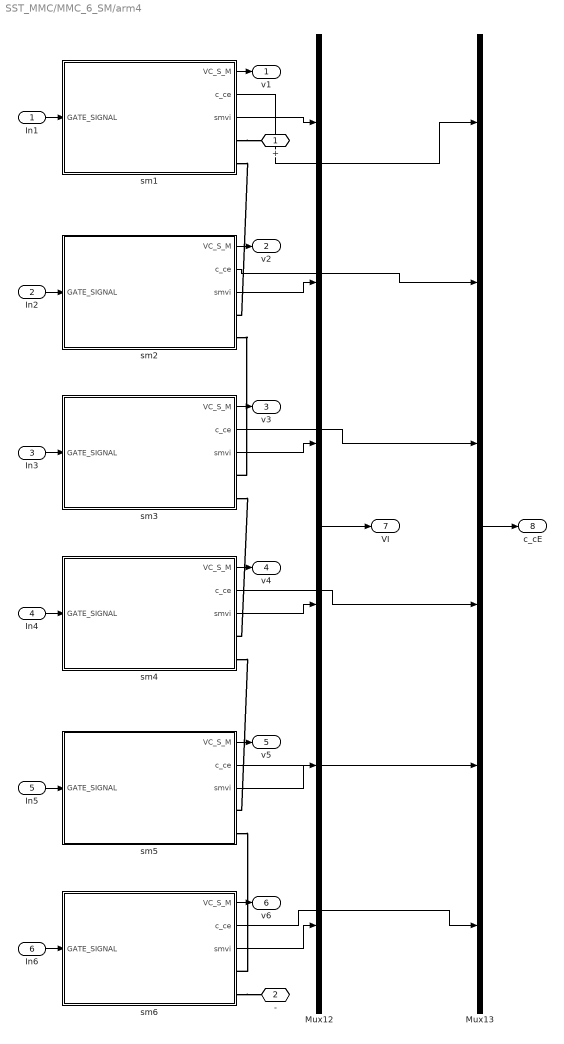
== system SST_MMC/MMC_6_SM/arm4 ==
  In1 : Inport
  In2 : Inport  Port=2
  In3 : Inport  Port=3
  In4 : Inport  Port=4
  In5 : Inport  Port=5
  In6 : Inport  Port=6
  Mux12 : Mux  Inputs=6
  Mux13 : Mux  Inputs=6
  sm1 : Subsystem
  sm2 : Subsystem
  sm3 : Subsystem
  sm4 : Subsystem
  sm5 : Subsystem
  sm6 : Subsystem
  + : PMIOPort  Port=1  Side=Right
  - : PMIOPort  Port=2  Side=Right
  v1 : Outport
  v2 : Outport  Port=2
  v3 : Outport  Port=3
  v4 : Outport  Port=4
  v5 : Outport  Port=5
  v6 : Outport  Port=6
  VI : Outport  Port=7
  c_cE : Outport  Port=8
  wires:
  sm1/3(" smvi") -> Mux12/1
  sm6/2(" c_ce") -> Mux13/6
  sm3/3(" smvi") -> Mux12/3
  sm2/2(" c_ce") -> Mux13/2
  sm1/2(" c_ce") -> Mux13/1
  sm3/2(" c_ce") -> Mux13/3
  sm6/3(" smvi") -> Mux12/6
  sm5/2(" c_ce") -> Mux13/5
  Mux12/1 -> VI/1
  sm4/1(" VC_S_M") -> v4/1
  sm1/1(" VC_S_M") -> v1/1
  sm4/3(" smvi") -> Mux12/4
  In6/1 -> sm6/1(" GATE_SIGNAL ")
  sm2/1(" VC_S_M") -> v2/1
  In1/1 -> sm1/1(" GATE_SIGNAL ")
  sm2/3(" smvi") -> Mux12/2
  In2/1 -> sm2/1(" GATE_SIGNAL ")
  sm6/1(" VC_S_M") -> v6/1
  In3/1 -> sm3/1(" GATE_SIGNAL ")
  sm5/1(" VC_S_M") -> v5/1
  In4/1 -> sm4/1(" GATE_SIGNAL ")
  In5/1 -> sm5/1(" GATE_SIGNAL ")
  Mux13/1 -> c_cE/1
  sm3/1(" VC_S_M") -> v3/1
  sm5/3(" smvi") -> Mux12/5
  sm4/2(" c_ce") -> Mux13/4
  connections:
  sm3/RConn2 -- sm4/RConn1
  sm5/RConn2 -- sm6/RConn1
  sm4/RConn2 -- sm5/RConn1
  sm2/RConn2 -- sm3/RConn1
  sm1/RConn1 -- +/RConn1
  sm1/RConn2 -- sm2/RConn1
  sm6/RConn2 -- -/RConn1

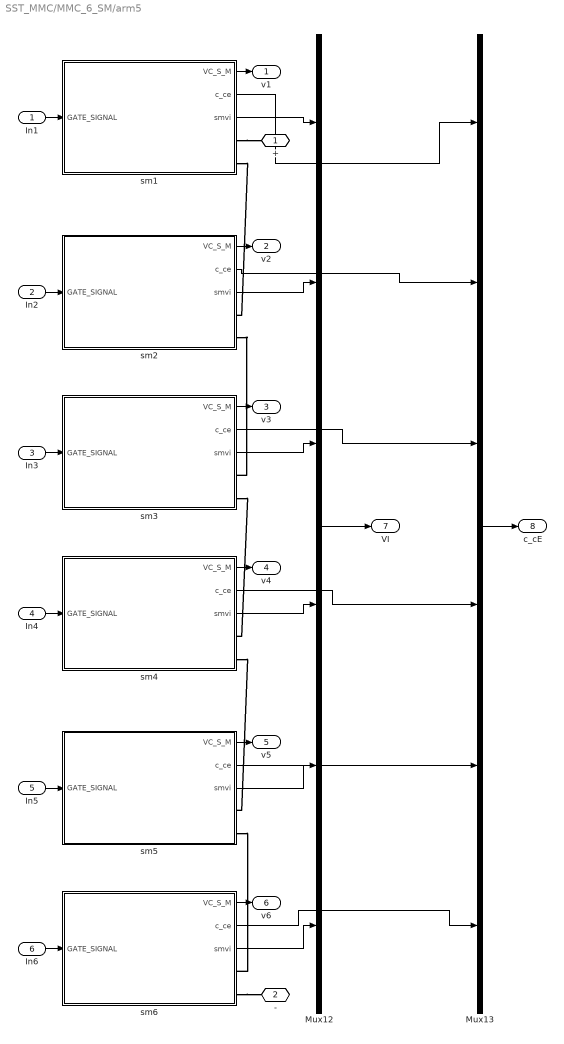
== system SST_MMC/MMC_6_SM/arm5 ==
  In1 : Inport
  In2 : Inport  Port=2
  In3 : Inport  Port=3
  In4 : Inport  Port=4
  In5 : Inport  Port=5
  In6 : Inport  Port=6
  Mux12 : Mux  Inputs=6
  Mux13 : Mux  Inputs=6
  sm1 : Subsystem
  sm2 : Subsystem
  sm3 : Subsystem
  sm4 : Subsystem
  sm5 : Subsystem
  sm6 : Subsystem
  + : PMIOPort  Port=1  Side=Right
  - : PMIOPort  Port=2  Side=Right
  v1 : Outport
  v2 : Outport  Port=2
  v3 : Outport  Port=3
  v4 : Outport  Port=4
  v5 : Outport  Port=5
  v6 : Outport  Port=6
  VI : Outport  Port=7
  c_cE : Outport  Port=8
  wires:
  sm4/2(" c_ce") -> Mux13/4
  sm5/3(" smvi") -> Mux12/5
  sm3/1(" VC_S_M") -> v3/1
  Mux13/1 -> c_cE/1
  In5/1 -> sm5/1(" GATE_SIGNAL ")
  In4/1 -> sm4/1(" GATE_SIGNAL ")
  sm5/1(" VC_S_M") -> v5/1
  In3/1 -> sm3/1(" GATE_SIGNAL ")
  sm6/1(" VC_S_M") -> v6/1
  In2/1 -> sm2/1(" GATE_SIGNAL ")
  sm2/3(" smvi") -> Mux12/2
  In1/1 -> sm1/1(" GATE_SIGNAL ")
  sm2/1(" VC_S_M") -> v2/1
  In6/1 -> sm6/1(" GATE_SIGNAL ")
  sm4/3(" smvi") -> Mux12/4
  sm1/1(" VC_S_M") -> v1/1
  sm4/1(" VC_S_M") -> v4/1
  Mux12/1 -> VI/1
  sm5/2(" c_ce") -> Mux13/5
  sm6/3(" smvi") -> Mux12/6
  sm3/2(" c_ce") -> Mux13/3
  sm1/2(" c_ce") -> Mux13/1
  sm2/2(" c_ce") -> Mux13/2
  sm3/3(" smvi") -> Mux12/3
  sm6/2(" c_ce") -> Mux13/6
  sm1/3(" smvi") -> Mux12/1
  connections:
  sm6/RConn2 -- -/RConn1
  sm1/RConn2 -- sm2/RConn1
  sm1/RConn1 -- +/RConn1
  sm2/RConn2 -- sm3/RConn1
  sm4/RConn2 -- sm5/RConn1
  sm5/RConn2 -- sm6/RConn1
  sm3/RConn2 -- sm4/RConn1

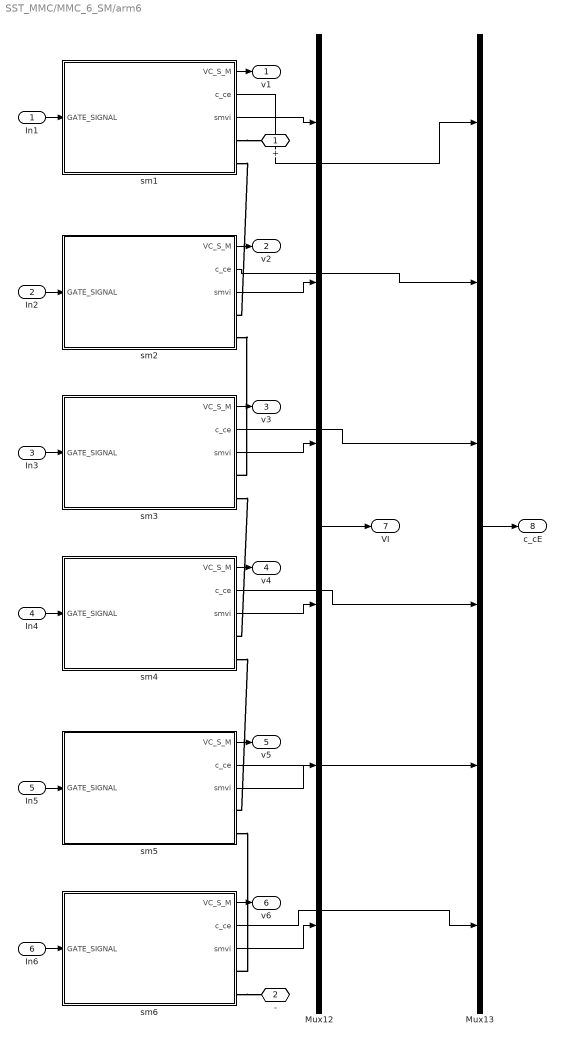
== system SST_MMC/MMC_6_SM/arm6 ==
  In1 : Inport
  In2 : Inport  Port=2
  In3 : Inport  Port=3
  In4 : Inport  Port=4
  In5 : Inport  Port=5
  In6 : Inport  Port=6
  Mux12 : Mux  Inputs=6
  Mux13 : Mux  Inputs=6
  sm1 : Subsystem
  sm2 : Subsystem
  sm3 : Subsystem
  sm4 : Subsystem
  sm5 : Subsystem
  sm6 : Subsystem
  + : PMIOPort  Port=1  Side=Right
  - : PMIOPort  Port=2  Side=Right
  v1 : Outport
  v2 : Outport  Port=2
  v3 : Outport  Port=3
  v4 : Outport  Port=4
  v5 : Outport  Port=5
  v6 : Outport  Port=6
  VI : Outport  Port=7
  c_cE : Outport  Port=8
  wires:
  sm1/3(" smvi") -> Mux12/1
  sm6/2(" c_ce") -> Mux13/6
  sm3/3(" smvi") -> Mux12/3
  sm2/2(" c_ce") -> Mux13/2
  sm1/2(" c_ce") -> Mux13/1
  sm3/2(" c_ce") -> Mux13/3
  sm6/3(" smvi") -> Mux12/6
  sm5/2(" c_ce") -> Mux13/5
  Mux12/1 -> VI/1
  sm4/1(" VC_S_M") -> v4/1
  sm1/1(" VC_S_M") -> v1/1
  sm4/3(" smvi") -> Mux12/4
  In6/1 -> sm6/1(" GATE_SIGNAL ")
  sm2/1(" VC_S_M") -> v2/1
  In1/1 -> sm1/1(" GATE_SIGNAL ")
  sm2/3(" smvi") -> Mux12/2
  In2/1 -> sm2/1(" GATE_SIGNAL ")
  sm6/1(" VC_S_M") -> v6/1
  In3/1 -> sm3/1(" GATE_SIGNAL ")
  sm5/1(" VC_S_M") -> v5/1
  In4/1 -> sm4/1(" GATE_SIGNAL ")
  In5/1 -> sm5/1(" GATE_SIGNAL ")
  Mux13/1 -> c_cE/1
  sm3/1(" VC_S_M") -> v3/1
  sm5/3(" smvi") -> Mux12/5
  sm4/2(" c_ce") -> Mux13/4
  connections:
  sm3/RConn2 -- sm4/RConn1
  sm5/RConn2 -- sm6/RConn1
  sm4/RConn2 -- sm5/RConn1
  sm2/RConn2 -- sm3/RConn1
  sm1/RConn1 -- +/RConn1
  sm1/RConn2 -- sm2/RConn1
  sm6/RConn2 -- -/RConn1

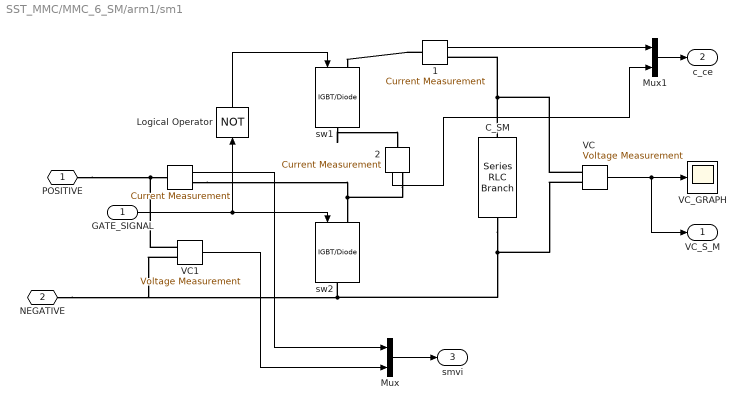
== system SST_MMC/MMC_6_SM/arm1/sm1 ==
  " GATE_SIGNAL " : Inport
  " " : powerlib/Measurements/Current Measurement  PhasorSimulation=off  OutputType=Complex  PSBequivalent=0
  " 1" : powerlib/Measurements/Current Measurement  PhasorSimulation=off  OutputType=Complex  PSBequivalent=0
  " 2" : powerlib/Measurements/Current Measurement  PhasorSimulation=off  OutputType=Complex  PSBequivalent=0
  C_SM : powerlib/Elements/Series RLC Branch  LConnTagsString=__new0  RConnTagsString=__new0  BranchType=C  Resistance=1  Inductance=1e-3  SetiL0=off  InitialCurrent=0  Capacitance=C_SM  Setx0=on  InitialVoltage=VC_SM  Measurements=None
  Logical Operator : Logic  Operator=NOT  AllPortsSameDT=off  OutDataTypeStr=boolean
  Mux : Mux  Inputs=2
  Mux1 : Mux  Inputs=2
  VC : powerlib/Measurements/Voltage Measurement  PhasorSimulation=off  OutputType=Complex  PSBequivalent=0
  VC1 : powerlib/Measurements/Voltage Measurement  PhasorSimulation=off  OutputType=Complex  PSBequivalent=0
  VC_GRAPH : Scope
      settings: YMin=150  YMax=1250
  sw1 : powerlib/Power Electronics/IGBT//Diode  Ron=Ron  Rs=1e5  Cs=inf  Measurements=off
  sw2 : powerlib/Power Electronics/IGBT//Diode  Ron=Ron  Rs=1e5  Cs=inf  Measurements=off
  POSITIVE : PMIOPort  Port=1  Side=Right
  NEGATIVE : PMIOPort  Port=2  Side=Right
  " VC_S_M" : Outport
  " c_ce" : Outport  Port=2
  " smvi" : Outport  Port=3
  wires:
  VC/1 -> " VC_S_M"/1, VC_GRAPH/1
  Logical Operator/1 -> sw1/1
  " GATE_SIGNAL "/1 -> Logical Operator/1, sw2/1
  " 1"/1 -> Mux1/1
  " 2"/1 -> Mux1/2
  " "/1 -> Mux/1
  VC1/1 -> Mux/2
  Mux1/1 -> " c_ce"/1
  Mux/1 -> " smvi"/1
  connections:
  sw1/RConn1 -- " 2"/LConn1
  VC/LConn2 -- C_SM/RConn1 -- VC1/LConn2 -- NEGATIVE/RConn1 -- sw2/RConn1
  VC/LConn1 -- C_SM/LConn1 -- " 1"/RConn1
  POSITIVE/RConn1 -- VC1/LConn1 -- " "/LConn1
  " 1"/LConn1 -- sw1/LConn1
  " 2"/RConn1 -- " "/RConn1 -- sw2/LConn1

== system SST_MMC/MMC_6_SM/arm1/sm2 ==
  " GATE_SIGNAL " : Inport
  " " : powerlib/Measurements/Current Measurement  PhasorSimulation=off  OutputType=Complex  PSBequivalent=0
  " 1" : powerlib/Measurements/Current Measurement  PhasorSimulation=off  OutputType=Complex  PSBequivalent=0
  " 2" : powerlib/Measurements/Current Measurement  PhasorSimulation=off  OutputType=Complex  PSBequivalent=0
  C_SM : powerlib/Elements/Series RLC Branch  LConnTagsString=__new0  RConnTagsString=__new0  BranchType=C  Resistance=1  Inductance=1e-3  SetiL0=off  InitialCurrent=0  Capacitance=C_SM  Setx0=on  InitialVoltage=VC_SM  Measurements=None
  Logical Operator : Logic  Operator=NOT  AllPortsSameDT=off  OutDataTypeStr=boolean
  Mux : Mux  Inputs=2
  Mux1 : Mux  Inputs=2
  VC : powerlib/Measurements/Voltage Measurement  PhasorSimulation=off  OutputType=Complex  PSBequivalent=0
  VC1 : powerlib/Measurements/Voltage Measurement  PhasorSimulation=off  OutputType=Complex  PSBequivalent=0
  VC_GRAPH : Scope
  sw1 : powerlib/Power Electronics/IGBT//Diode  Ron=Ron  Rs=1e5  Cs=inf  Measurements=off
  sw2 : powerlib/Power Electronics/IGBT//Diode  Ron=Ron  Rs=1e5  Cs=inf  Measurements=off
  POSITIVE : PMIOPort  Port=1  Side=Right
  NEGATIVE : PMIOPort  Port=2  Side=Right
  " VC_S_M" : Outport
  " c_ce" : Outport  Port=2
  " smvi" : Outport  Port=3
  wires:
  Mux/1 -> " smvi"/1
  Mux1/1 -> " c_ce"/1
  VC1/1 -> Mux/2
  " "/1 -> Mux/1
  " 2"/1 -> Mux1/2
  " 1"/1 -> Mux1/1
  " GATE_SIGNAL "/1 -> sw2/1, Logical Operator/1
  Logical Operator/1 -> sw1/1
  VC/1 -> VC_GRAPH/1, " VC_S_M"/1
  connections:
  " "/RConn1 -- sw2/LConn1 -- " 2"/RConn1
  " 1"/LConn1 -- sw1/LConn1
  VC1/LConn1 -- " "/LConn1 -- POSITIVE/RConn1
  " 1"/RConn1 -- C_SM/LConn1 -- VC/LConn1
  VC1/LConn2 -- NEGATIVE/RConn1 -- sw2/RConn1 -- C_SM/RConn1 -- VC/LConn2
  sw1/RConn1 -- " 2"/LConn1

== system SST_MMC/MMC_6_SM/arm1/sm3 ==
  " GATE_SIGNAL " : Inport
  " " : powerlib/Measurements/Current Measurement  PhasorSimulation=off  OutputType=Complex  PSBequivalent=0
  " 1" : powerlib/Measurements/Current Measurement  PhasorSimulation=off  OutputType=Complex  PSBequivalent=0
  " 2" : powerlib/Measurements/Current Measurement  PhasorSimulation=off  OutputType=Complex  PSBequivalent=0
  C_SM : powerlib/Elements/Series RLC Branch  LConnTagsString=__new0  RConnTagsString=__new0  BranchType=C  Resistance=1  Inductance=1e-3  SetiL0=off  InitialCurrent=0  Capacitance=C_SM  Setx0=on  InitialVoltage=VC_SM  Measurements=None
  Logical Operator : Logic  Operator=NOT  AllPortsSameDT=off  OutDataTypeStr=boolean
  Mux : Mux  Inputs=2
  Mux1 : Mux  Inputs=2
  VC : powerlib/Measurements/Voltage Measurement  PhasorSimulation=off  OutputType=Complex  PSBequivalent=0
  VC1 : powerlib/Measurements/Voltage Measurement  PhasorSimulation=off  OutputType=Complex  PSBequivalent=0
  VC_GRAPH : Scope
  sw1 : powerlib/Power Electronics/IGBT//Diode  Ron=Ron  Rs=1e5  Cs=inf  Measurements=off
  sw2 : powerlib/Power Electronics/IGBT//Diode  Ron=Ron  Rs=1e5  Cs=inf  Measurements=off
  POSITIVE : PMIOPort  Port=1  Side=Right
  NEGATIVE : PMIOPort  Port=2  Side=Right
  " VC_S_M" : Outport
  " c_ce" : Outport  Port=2
  " smvi" : Outport  Port=3
  wires:
  VC/1 -> " VC_S_M"/1, VC_GRAPH/1
  Logical Operator/1 -> sw1/1
  " GATE_SIGNAL "/1 -> Logical Operator/1, sw2/1
  " 1"/1 -> Mux1/1
  " 2"/1 -> Mux1/2
  " "/1 -> Mux/1
  VC1/1 -> Mux/2
  Mux1/1 -> " c_ce"/1
  Mux/1 -> " smvi"/1
  connections:
  sw1/RConn1 -- " 2"/LConn1
  VC/LConn2 -- C_SM/RConn1 -- sw2/RConn1 -- NEGATIVE/RConn1 -- VC1/LConn2
  VC/LConn1 -- C_SM/LConn1 -- " 1"/RConn1
  POSITIVE/RConn1 -- " "/LConn1 -- VC1/LConn1
  " 1"/LConn1 -- sw1/LConn1
  " 2"/RConn1 -- sw2/LConn1 -- " "/RConn1

== system SST_MMC/MMC_6_SM/arm1/sm4 ==
  " GATE_SIGNAL " : Inport
  " " : powerlib/Measurements/Current Measurement  PhasorSimulation=off  OutputType=Complex  PSBequivalent=0
  " 1" : powerlib/Measurements/Current Measurement  PhasorSimulation=off  OutputType=Complex  PSBequivalent=0
  " 2" : powerlib/Measurements/Current Measurement  PhasorSimulation=off  OutputType=Complex  PSBequivalent=0
  C_SM : powerlib/Elements/Series RLC Branch  LConnTagsString=__new0  RConnTagsString=__new0  BranchType=C  Resistance=1  Inductance=1e-3  SetiL0=off  InitialCurrent=0  Capacitance=C_SM  Setx0=on  InitialVoltage=VC_SM  Measurements=None
  Logical Operator : Logic  Operator=NOT  AllPortsSameDT=off  OutDataTypeStr=boolean
  Mux : Mux  Inputs=2
  Mux1 : Mux  Inputs=2
  VC : powerlib/Measurements/Voltage Measurement  PhasorSimulation=off  OutputType=Complex  PSBequivalent=0
  VC1 : powerlib/Measurements/Voltage Measurement  PhasorSimulation=off  OutputType=Complex  PSBequivalent=0
  VC_GRAPH : Scope
  sw1 : powerlib/Power Electronics/IGBT//Diode  Ron=Ron  Rs=1e5  Cs=inf  Measurements=off
  sw2 : powerlib/Power Electronics/IGBT//Diode  Ron=Ron  Rs=1e5  Cs=inf  Measurements=off
  POSITIVE : PMIOPort  Port=1  Side=Right
  NEGATIVE : PMIOPort  Port=2  Side=Right
  " VC_S_M" : Outport
  " c_ce" : Outport  Port=2
  " smvi" : Outport  Port=3
  wires:
  Mux/1 -> " smvi"/1
  Mux1/1 -> " c_ce"/1
  VC1/1 -> Mux/2
  " "/1 -> Mux/1
  " 2"/1 -> Mux1/2
  " 1"/1 -> Mux1/1
  " GATE_SIGNAL "/1 -> sw2/1, Logical Operator/1
  Logical Operator/1 -> sw1/1
  VC/1 -> VC_GRAPH/1, " VC_S_M"/1
  connections:
  " "/RConn1 -- sw2/LConn1 -- " 2"/RConn1
  " 1"/LConn1 -- sw1/LConn1
  VC1/LConn1 -- " "/LConn1 -- POSITIVE/RConn1
  " 1"/RConn1 -- C_SM/LConn1 -- VC/LConn1
  VC1/LConn2 -- NEGATIVE/RConn1 -- sw2/RConn1 -- C_SM/RConn1 -- VC/LConn2
  sw1/RConn1 -- " 2"/LConn1

== system SST_MMC/MMC_6_SM/arm1/sm5 ==
  " GATE_SIGNAL " : Inport
  " " : powerlib/Measurements/Current Measurement  PhasorSimulation=off  OutputType=Complex  PSBequivalent=0
  " 1" : powerlib/Measurements/Current Measurement  PhasorSimulation=off  OutputType=Complex  PSBequivalent=0
  " 2" : powerlib/Measurements/Current Measurement  PhasorSimulation=off  OutputType=Complex  PSBequivalent=0
  C_SM : powerlib/Elements/Series RLC Branch  LConnTagsString=__new0  RConnTagsString=__new0  BranchType=C  Resistance=1  Inductance=1e-3  SetiL0=off  InitialCurrent=0  Capacitance=C_SM  Setx0=on  InitialVoltage=VC_SM  Measurements=None
  Logical Operator : Logic  Operator=NOT  AllPortsSameDT=off  OutDataTypeStr=boolean
  Mux : Mux  Inputs=2
  Mux1 : Mux  Inputs=2
  VC : powerlib/Measurements/Voltage Measurement  PhasorSimulation=off  OutputType=Complex  PSBequivalent=0
  VC1 : powerlib/Measurements/Voltage Measurement  PhasorSimulation=off  OutputType=Complex  PSBequivalent=0
  VC_GRAPH : Scope
  sw1 : powerlib/Power Electronics/IGBT//Diode  Ron=Ron  Rs=1e5  Cs=inf  Measurements=off
  sw2 : powerlib/Power Electronics/IGBT//Diode  Ron=Ron  Rs=1e5  Cs=inf  Measurements=off
  POSITIVE : PMIOPort  Port=1  Side=Right
  NEGATIVE : PMIOPort  Port=2  Side=Right
  " VC_S_M" : Outport
  " c_ce" : Outport  Port=2
  " smvi" : Outport  Port=3
  wires:
  VC/1 -> " VC_S_M"/1, VC_GRAPH/1
  Logical Operator/1 -> sw1/1
  " GATE_SIGNAL "/1 -> Logical Operator/1, sw2/1
  " 1"/1 -> Mux1/1
  " 2"/1 -> Mux1/2
  " "/1 -> Mux/1
  VC1/1 -> Mux/2
  Mux1/1 -> " c_ce"/1
  Mux/1 -> " smvi"/1
  connections:
  sw1/RConn1 -- " 2"/LConn1
  VC/LConn2 -- C_SM/RConn1 -- sw2/RConn1 -- NEGATIVE/RConn1 -- VC1/LConn2
  VC/LConn1 -- C_SM/LConn1 -- " 1"/RConn1
  POSITIVE/RConn1 -- " "/LConn1 -- VC1/LConn1
  " 1"/LConn1 -- sw1/LConn1
  " 2"/RConn1 -- sw2/LConn1 -- " "/RConn1

== system SST_MMC/MMC_6_SM/arm1/sm6 ==
  " GATE_SIGNAL " : Inport
  " " : powerlib/Measurements/Current Measurement  PhasorSimulation=off  OutputType=Complex  PSBequivalent=0
  " 1" : powerlib/Measurements/Current Measurement  PhasorSimulation=off  OutputType=Complex  PSBequivalent=0
  " 2" : powerlib/Measurements/Current Measurement  PhasorSimulation=off  OutputType=Complex  PSBequivalent=0
  C_SM : powerlib/Elements/Series RLC Branch  LConnTagsString=__new0  RConnTagsString=__new0  BranchType=C  Resistance=1  Inductance=1e-3  SetiL0=off  InitialCurrent=0  Capacitance=C_SM  Setx0=on  InitialVoltage=VC_SM  Measurements=None
  Logical Operator : Logic  Operator=NOT  AllPortsSameDT=off  OutDataTypeStr=boolean
  Mux : Mux  Inputs=2
  Mux1 : Mux  Inputs=2
  VC : powerlib/Measurements/Voltage Measurement  PhasorSimulation=off  OutputType=Complex  PSBequivalent=0
  VC1 : powerlib/Measurements/Voltage Measurement  PhasorSimulation=off  OutputType=Complex  PSBequivalent=0
  VC_GRAPH : Scope
  sw1 : powerlib/Power Electronics/IGBT//Diode  Ron=Ron  Rs=1e5  Cs=inf  Measurements=off
  sw2 : powerlib/Power Electronics/IGBT//Diode  Ron=Ron  Rs=1e5  Cs=inf  Measurements=off
  POSITIVE : PMIOPort  Port=1  Side=Right
  NEGATIVE : PMIOPort  Port=2  Side=Right
  " VC_S_M" : Outport
  " c_ce" : Outport  Port=2
  " smvi" : Outport  Port=3
  wires:
  Mux/1 -> " smvi"/1
  Mux1/1 -> " c_ce"/1
  VC1/1 -> Mux/2
  " "/1 -> Mux/1
  " 2"/1 -> Mux1/2
  " 1"/1 -> Mux1/1
  " GATE_SIGNAL "/1 -> sw2/1, Logical Operator/1
  Logical Operator/1 -> sw1/1
  VC/1 -> VC_GRAPH/1, " VC_S_M"/1
  connections:
  " "/RConn1 -- sw2/LConn1 -- " 2"/RConn1
  " 1"/LConn1 -- sw1/LConn1
  VC1/LConn1 -- " "/LConn1 -- POSITIVE/RConn1
  " 1"/RConn1 -- C_SM/LConn1 -- VC/LConn1
  VC1/LConn2 -- NEGATIVE/RConn1 -- sw2/RConn1 -- C_SM/RConn1 -- VC/LConn2
  sw1/RConn1 -- " 2"/LConn1

== system SST_MMC/MMC_6_SM/arm2/sm1 ==
  " GATE_SIGNAL " : Inport
  " " : powerlib/Measurements/Current Measurement  PhasorSimulation=off  OutputType=Complex  PSBequivalent=0
  " 1" : powerlib/Measurements/Current Measurement  PhasorSimulation=off  OutputType=Complex  PSBequivalent=0
  " 2" : powerlib/Measurements/Current Measurement  PhasorSimulation=off  OutputType=Complex  PSBequivalent=0
  C_SM : powerlib/Elements/Series RLC Branch  LConnTagsString=__new0  RConnTagsString=__new0  BranchType=C  Resistance=1  Inductance=1e-3  SetiL0=off  InitialCurrent=0  Capacitance=C_SM  Setx0=on  InitialVoltage=VC_SM  Measurements=None
  Logical Operator : Logic  Operator=NOT  AllPortsSameDT=off  OutDataTypeStr=boolean
  Mux : Mux  Inputs=2
  Mux1 : Mux  Inputs=2
  VC : powerlib/Measurements/Voltage Measurement  PhasorSimulation=off  OutputType=Complex  PSBequivalent=0
  VC1 : powerlib/Measurements/Voltage Measurement  PhasorSimulation=off  OutputType=Complex  PSBequivalent=0
  VC_GRAPH : Scope
  sw1 : powerlib/Power Electronics/IGBT//Diode  Ron=Ron  Rs=1e5  Cs=inf  Measurements=off
  sw2 : powerlib/Power Electronics/IGBT//Diode  Ron=Ron  Rs=1e5  Cs=inf  Measurements=off
  POSITIVE : PMIOPort  Port=1  Side=Right
  NEGATIVE : PMIOPort  Port=2  Side=Right
  " VC_S_M" : Outport
  " c_ce" : Outport  Port=2
  " smvi" : Outport  Port=3
  wires:
  Mux/1 -> " smvi"/1
  Mux1/1 -> " c_ce"/1
  VC1/1 -> Mux/2
  " "/1 -> Mux/1
  " 2"/1 -> Mux1/2
  " 1"/1 -> Mux1/1
  " GATE_SIGNAL "/1 -> sw2/1, Logical Operator/1
  Logical Operator/1 -> sw1/1
  VC/1 -> VC_GRAPH/1, " VC_S_M"/1
  connections:
  " "/RConn1 -- sw2/LConn1 -- " 2"/RConn1
  " 1"/LConn1 -- sw1/LConn1
  VC1/LConn1 -- " "/LConn1 -- POSITIVE/RConn1
  " 1"/RConn1 -- C_SM/LConn1 -- VC/LConn1
  VC1/LConn2 -- NEGATIVE/RConn1 -- sw2/RConn1 -- C_SM/RConn1 -- VC/LConn2
  sw1/RConn1 -- " 2"/LConn1

== system SST_MMC/MMC_6_SM/arm2/sm2 ==
  " GATE_SIGNAL " : Inport
  " " : powerlib/Measurements/Current Measurement  PhasorSimulation=off  OutputType=Complex  PSBequivalent=0
  " 1" : powerlib/Measurements/Current Measurement  PhasorSimulation=off  OutputType=Complex  PSBequivalent=0
  " 2" : powerlib/Measurements/Current Measurement  PhasorSimulation=off  OutputType=Complex  PSBequivalent=0
  C_SM : powerlib/Elements/Series RLC Branch  LConnTagsString=__new0  RConnTagsString=__new0  BranchType=C  Resistance=1  Inductance=1e-3  SetiL0=off  InitialCurrent=0  Capacitance=C_SM  Setx0=on  InitialVoltage=VC_SM  Measurements=None
  Logical Operator : Logic  Operator=NOT  AllPortsSameDT=off  OutDataTypeStr=boolean
  Mux : Mux  Inputs=2
  Mux1 : Mux  Inputs=2
  VC : powerlib/Measurements/Voltage Measurement  PhasorSimulation=off  OutputType=Complex  PSBequivalent=0
  VC1 : powerlib/Measurements/Voltage Measurement  PhasorSimulation=off  OutputType=Complex  PSBequivalent=0
  VC_GRAPH : Scope
  sw1 : powerlib/Power Electronics/IGBT//Diode  Ron=Ron  Rs=1e5  Cs=inf  Measurements=off
  sw2 : powerlib/Power Electronics/IGBT//Diode  Ron=Ron  Rs=1e5  Cs=inf  Measurements=off
  POSITIVE : PMIOPort  Port=1  Side=Right
  NEGATIVE : PMIOPort  Port=2  Side=Right
  " VC_S_M" : Outport
  " c_ce" : Outport  Port=2
  " smvi" : Outport  Port=3
  wires:
  VC/1 -> " VC_S_M"/1, VC_GRAPH/1
  Logical Operator/1 -> sw1/1
  " GATE_SIGNAL "/1 -> Logical Operator/1, sw2/1
  " 1"/1 -> Mux1/1
  " 2"/1 -> Mux1/2
  " "/1 -> Mux/1
  VC1/1 -> Mux/2
  Mux1/1 -> " c_ce"/1
  Mux/1 -> " smvi"/1
  connections:
  sw1/RConn1 -- " 2"/LConn1
  VC/LConn2 -- C_SM/RConn1 -- sw2/RConn1 -- NEGATIVE/RConn1 -- VC1/LConn2
  VC/LConn1 -- C_SM/LConn1 -- " 1"/RConn1
  POSITIVE/RConn1 -- " "/LConn1 -- VC1/LConn1
  " 1"/LConn1 -- sw1/LConn1
  " 2"/RConn1 -- sw2/LConn1 -- " "/RConn1

== system SST_MMC/MMC_6_SM/arm2/sm3 ==
  " GATE_SIGNAL " : Inport
  " " : powerlib/Measurements/Current Measurement  PhasorSimulation=off  OutputType=Complex  PSBequivalent=0
  " 1" : powerlib/Measurements/Current Measurement  PhasorSimulation=off  OutputType=Complex  PSBequivalent=0
  " 2" : powerlib/Measurements/Current Measurement  PhasorSimulation=off  OutputType=Complex  PSBequivalent=0
  C_SM : powerlib/Elements/Series RLC Branch  LConnTagsString=__new0  RConnTagsString=__new0  BranchType=C  Resistance=1  Inductance=1e-3  SetiL0=off  InitialCurrent=0  Capacitance=C_SM  Setx0=on  InitialVoltage=VC_SM  Measurements=None
  Logical Operator : Logic  Operator=NOT  AllPortsSameDT=off  OutDataTypeStr=boolean
  Mux : Mux  Inputs=2
  Mux1 : Mux  Inputs=2
  VC : powerlib/Measurements/Voltage Measurement  PhasorSimulation=off  OutputType=Complex  PSBequivalent=0
  VC1 : powerlib/Measurements/Voltage Measurement  PhasorSimulation=off  OutputType=Complex  PSBequivalent=0
  VC_GRAPH : Scope
  sw1 : powerlib/Power Electronics/IGBT//Diode  Ron=Ron  Rs=1e5  Cs=inf  Measurements=off
  sw2 : powerlib/Power Electronics/IGBT//Diode  Ron=Ron  Rs=1e5  Cs=inf  Measurements=off
  POSITIVE : PMIOPort  Port=1  Side=Right
  NEGATIVE : PMIOPort  Port=2  Side=Right
  " VC_S_M" : Outport
  " c_ce" : Outport  Port=2
  " smvi" : Outport  Port=3
  wires:
  Mux/1 -> " smvi"/1
  Mux1/1 -> " c_ce"/1
  VC1/1 -> Mux/2
  " "/1 -> Mux/1
  " 2"/1 -> Mux1/2
  " 1"/1 -> Mux1/1
  " GATE_SIGNAL "/1 -> sw2/1, Logical Operator/1
  Logical Operator/1 -> sw1/1
  VC/1 -> VC_GRAPH/1, " VC_S_M"/1
  connections:
  " "/RConn1 -- sw2/LConn1 -- " 2"/RConn1
  " 1"/LConn1 -- sw1/LConn1
  VC1/LConn1 -- " "/LConn1 -- POSITIVE/RConn1
  " 1"/RConn1 -- C_SM/LConn1 -- VC/LConn1
  VC1/LConn2 -- NEGATIVE/RConn1 -- sw2/RConn1 -- C_SM/RConn1 -- VC/LConn2
  sw1/RConn1 -- " 2"/LConn1
